simulink model "old_matlab_fnc"  (R2020a)
settings: Solver=VariableStepAuto  StartTime=0.0  StopTime=10.0  RelTol=1e-3
values from neighbouring files (symbols this model uses):
  Ts = 0.1    [main_adaptive_mpc.m]
  Xi = zeros(1,nX)    [GetAuvSimAndJacobian.m]    (also in main_adaptive_mpc.m = [0;0;0;0;0;0;0;0;0;0;0;0])
settings Model: Creator=lamarre  LastModifiedBy=lamarre

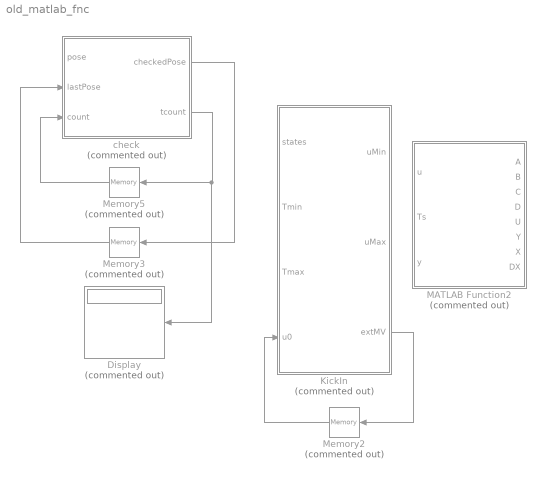
== system old_matlab_fnc ==
  Display : Display  Commented=on
  KickIn : MATLAB Function  Commented=on  TreatAsAtomicUnit=on  SystemSampleTime=Ts
  MATLAB Function2 : MATLAB Function  Commented=on  TreatAsAtomicUnit=on  SystemSampleTime=Ts
  Memory2 : Memory  Commented=on  InitialCondition=[0;0;0;0;-7.1;6.94;-7.49;7.65]
  Memory3 : Memory  Commented=on  InitialCondition=Xi
  Memory5 : Memory  Commented=on  InitialCondition=[0,0,0]
  check : MATLAB Function  Commented=on  TreatAsAtomicUnit=on  SystemSampleTime=Ts
  wires:
  Memory2/1 -> KickIn/4(u0)
  Memory5/1 -> check/3(count)
  check/2(tcount) -> Display/1, Memory5/1
  check/1(checkedPose) -> Memory3/1
  Memory3/1 -> check/2(lastPose)
  KickIn/3(extMV) -> Memory2/1

== matlab function old_matlab_fnc/MATLAB Function2 ==
  data: u input; Ts input; y input; A output; B output; C output; D output; U output; Y output; X output; DX output
function [A,B,C,D,U,Y,X,DX] = TrimPlant(u,Ts,y)
% Lineariser le model dynamique

%x=[y(4:5,1);y(7:12,1)];
%x(5)=x(5)-.85;
tic;
[Ac, Bc, Cc, Dc]=AUVStateJacobianFcn(y,u);
% Generate discrete-time model

%  nx = size(Ac,1);
%  nu = size(Bc,2);
%cplant=ss(Ac,Bc,Cc,Dc);
%plant=c2d(cplant,Ts,'zoh');

nx = size(Ac,1);
nu = size(Bc,2);
M = expm([[Ac Bc]*Ts; zeros(nu,nu+nx)]);
A = M(1:nx,1:nx);
B = M(1:nx,nx+1:nx+nu);
C = Cc;
D = Dc;
 %xx=[X(4:5,1);X(7:12)];

% cplant=ss(Ac,Bc,Cc,Dc);
% plant=c2d(cplant,Ts,'zoh');
%plant=ss(A,B,C,D,Ts);

% Nominal conditions for discrete-time plant
U=u.';
Y=(Cc*y + Dc*u).';
X=y.';
DX=(A*y+B*u-y).';
toc;
end

== matlab function old_matlab_fnc/KickIn ==
  data: uMin output; uMax output; states input size=12; Tmin input; Tmax input; extMV output size=8; u0 input size=8
function [uMin,uMax,extMV] = KickIn(states,Tmin,Tmax,u0)

uMin=Tmin;
uMax=Tmax;

% Fonction objective.
fun = @(x)sum(abs(u0.'-x));

% Retrouver la matrice gravité et thruster
Aeq=ThrusterMatrix().';
Beq=Gravity(states).';

% Optimiser la commande pour la condition initial
op=optimoptions('fmincon','Algorithm','sqp','ConstraintTolerance',0.01,...
                'OptimalityTolerance',0.01);
            
extMV=-fmincon(fun,u0.',[],[],Aeq,Beq,[],[],[],op).';

% Calculer la nouvelle limite thruster
for i=1:size(extMV,1)
    if extMV(i)>0
        uMax(i)= uMax(i)-extMV(i);
    else
        uMin(i)= uMin(i)-extMV(i);
    end
end

== matlab function old_matlab_fnc/check ==
  data: pose input size=[12 1]; checkedPose output size=[12 1]; lastPose input size=[12 1]; count input size=3; tcount output
function[checkedPose,tcount]= discontinuityCheck(pose,lastPose,count)
           % Cette fonction vérifie et corrige au besoin la discontinuite
           % des angles de rotation.
           tcount=count;
           checkedPose=pose;
           
          for i=4:6 % compute roll pitch yaw
              
              % appliquer la discontinuté actuelle
               if tcount(i-3)>0
                   checkedPose(i)=(pose(i)+pi)+(pi*tcount(i-3));
               elseif tcount<0
                   checkedPose(i)=(pose(i)-pi)+(pi*tcount(i-3));
               end
               
               % calculer la différence entre 2 point
               delta=lastPose(i)-checkedPose(i);
              
               
               % Verifier la discontinuité de laxe
               if abs (delta)>=pi 
                   % Determiner le sens de la discontinuité
                   if delta >0 
                      % Ajouter un tour
                      tcount(i-3)=tcount(i-3)+1;
                      % Recaluler l'angle
                      if tcount(i-3)==0
                        checkedPose(i)=pose(i);
                      else
                        checkedPose(i)=(pi+pose(i))+(pi*tcount(i-3));
                      end
                   else
                      % Soustraire un tour
                      tcount(i-3)=tcount(i-3)-1;
                      % Recaluler l'angle
                      if tcount(i-3)==0
                        checkedPose(i)=pose(i);
                      else
                        checkedPose(i)=(pose(i)-pi)+(pi*tcount(i-3));
                      end
                   end
               end   
           end
end
